simulink model "player_ball_7_8players"  (R2021b)
settings: Solver=VariableStepAuto  StartTime=0.0  StopTime=300  RelTol=1e-3
model workspace (MAT data in the model file):
  trailfuzzy = 'trailfuzzy.fis'
values from neighbouring files (symbols this model uses):
  initBallPos = fieldCenter    [robotSoccerParams.m]
  robotDetectorMaxHits = 5    [robotSoccerParams.m]
  sampleTime = 0.05    [robotSoccerParams.m]
undefined symbols (not defined in the file or in its folder): DiscIntNeverNeededParam
libraries: mobileRoboticsLib x41, dspindex x14, fuzblock x8
(part 2 of 2)

== matlab function player_ball_7_8players/idx3 goal_range_angles ==
  data: u input; goalRight_angle output; goalRange output; goalLeft_angle output; rPose_x input; rPose_y input
% function y = fcn(u)
% for i = 1:5
%     if u(i,3) == 1
%         a = u(i,:)
%     end
% end
% % b = u(2,:)
% % c = u(3,:)
% % d = u(4,:)
% % e = u(5,:)
% y = a;
% end
%two indexes are same. How to identify right and left angles
% for now randomly assigned the values
% goal range is minimum of the two 


function [goalRight_angle,goalRange, goalLeft_angle]= fcn(u,rPose_x, rPose_y)
goalRight_angle=0;
goalLeft_angle=0;
right_range = 0;
left_range =0;

x=0;
%if rPose_y1> 15 &&  rPose_y1< 45 && rPose_theta1 > 0
leftPolePose = [90 45];
rightPolePose = [90 15];
robotPose = [rPose_x rPose_y];
rightPole_dist = norm(rightPolePose - robotPose);
leftPole_dist = norm(leftPolePose - robotPose);
if rightPole_dist< leftPole_dist
    k=0;
    for i= 1:5
        if u(i,3) == 3 && k==0
            goalRight_angle = u(i,2);
            right_range = u(i,1);
            k = k+1;
        elseif u(i,3) ==3 && k==1
            goalLeft_angle = u(i,2);
            left_range = u(i,1);
            k =0;

        end
    end
else
    k=0;
    for i= 1:5
        if u(i,3) == 3 && k==0
            goalLeft_angle = u(i,2);
            left_range = u(i,1);
            k = k+1;
        elseif u(i,3) ==3 && k==1
            goalRight_angle = u(i,2);
            right_range = u(i,1);
            k =0;

        end
    end
end

if right_range < left_range
    goalRange = right_range;
else
    goalRange = left_range;
end

== matlab function player_ball_7_8players/Zero Pad Detections4 ==
  data: u input size=[maxHits 3]; y output size=[maxHits 3]; maxHits parameter
function y = zeroPad(u,maxHits)
% Zero-pads object detections to work with arrays of buses

y = zeros(maxHits,3);
numElems = min(size(u,1),maxHits);
for idx = 1:numElems
   y(idx,1:3) = u(idx,1:3); 
end

== matlab function player_ball_7_8players/Ball Dynamics1 ==
  data: ballPose output; ballHeld input; KickPower input; rPose_x input; rPose_y input; rPose_theta input
function ballPose  = fcn(ballHeld, KickPower,rPose_x, rPose_y, rPose_theta)
ballPose = [25 10];
if ballHeld == 1 
    ballPose = [rPose_x rPose_y] + (0.8 + 0.3)*[cos(rPose_theta) sin(rPose_theta)];

elseif KickPower >= 5.5 && ballHeld == 1
    %ballPose = KickPower*[rPose_x rPose_y] + (0.8 + 0.3)*[cos(rPose_theta) sin(rPose_theta)];
    ballHeld = 0
    ballPose = KickPower*[rPose_x rPose_y] + (0.8 + 0.3)*[cos(rPose_theta) sin(rPose_theta)];
    %if KickPower ~=0
    %    ballPose = KickPower*[rPose_x rPose_y] + (0.8 + 0.3)*[cos(rPose_theta) sin(rPose_theta)];
    %end

end

== matlab function player_ball_7_8players/MATLAB Function1 ==
  data: u input; y output
function y = fcn(u)

if u > 3.15
    u = pi -(u - pi);
end

if u <-3.15
    u = pi + (u + pi);
end     

y = u;

== matlab function player_ball_7_8players/Zero Pad Detections1 ==
  data: u input size=[maxHits 3]; y output size=[maxHits 3]; maxHits parameter
function y = zeroPad(u,maxHits)
% Zero-pads object detections to work with arrays of buses

y = zeros(maxHits,3);
numElems = min(size(u,1),maxHits);
for idx = 1:numElems
   y(idx,1:3) = u(idx,1:3); 
end

== matlab function player_ball_7_8players/Zero Pad Detections5 ==
  data: u input size=[maxHits 3]; y output size=[maxHits 3]; maxHits parameter
function y = zeroPad(u,maxHits)
% Zero-pads object detections to work with arrays of buses

y = zeros(maxHits,3);
numElems = min(size(u,1),maxHits);
for idx = 1:numElems
   y(idx,1:3) = u(idx,1:3); 
end

== matlab function player_ball_7_8players/Zero Pad Detections6 ==
  data: u input size=[maxHits 3]; y output size=[maxHits 3]; maxHits parameter
function y = zeroPad(u,maxHits)
% Zero-pads object detections to work with arrays of buses

y = zeros(maxHits,3);
numElems = min(size(u,1),maxHits);
for idx = 1:numElems
   y(idx,1:3) = u(idx,1:3); 
end

== matlab function player_ball_7_8players/Zero Pad Detections7 ==
  data: u input size=[maxHits 3]; y output size=[maxHits 3]; maxHits parameter
function y = zeroPad(u,maxHits)
% Zero-pads object detections to work with arrays of buses

y = zeros(maxHits,3);
numElems = min(size(u,1),maxHits);
for idx = 1:numElems
   y(idx,1:3) = u(idx,1:3); 
end

== matlab function player_ball_7_8players/ball1 ==
  data: u input; y output; ballHeld output; robotIdx output; ballHeld input; robotIdx input

function [y,ballHeld, robotIdx]= fcn(u,ballHeld,robotIdx)
% a = u(1,:);
% b = u(2,:);
% c = u(3,:);
% d = u(4,:);
% e = u(5,:);
% robotIdx =2;
% if a(3) ==1
%     y = a;
% 
% 
% elseif b(3) ==1
%     y = b;
% 
% 
% elseif c(3)==1
%     y=c;
% 
% 
% elseif d(3)==1
%     y=d;
% 
% 
% else
%     y = e;
% 
% 
% end
% if y(1)  <= 1.1
%     ballHeld = 1;
%     %robotIdx =2;
% 
% else
%     ballHeld =0;
%     %robotIdx =0;
% 
% end
a = u(1,:);
b = u(2,:);
c = u(3,:);
d = u(4,:);
e = u(5,:);
robotIdx =2;
if a(3) ==1
    y = a;


elseif b(3) ==1
    y = b;


elseif c(3)==1
    y=c;


elseif d(3)==1
    y=d;


else
    y = e;


end
if y(1)  <= 1.1
    ballHeld = 1;
    %robotIdx =1;
    %possession = robotIdx;

else
    ballHeld =0;
    %robotIdx =0;

end

== matlab function player_ball_7_8players/idx3 goal_range_angles1 ==
  data: u input; goalRight_angle output; goalRange output; goalLeft_angle output; rPose_x input; rPose_y input
% function y = fcn(u)
% for i = 1:5
%     if u(i,3) == 1
%         a = u(i,:)
%     end
% end
% % b = u(2,:)
% % c = u(3,:)
% % d = u(4,:)
% % e = u(5,:)
% y = a;
% end
%two indexes are same. How to identify right and left angles
% for now randomly assigned the values
% goal range is minimum of the two 


function [goalRight_angle,goalRange, goalLeft_angle]= fcn(u,rPose_x,rPose_y)
goalRight_angle=0;
goalLeft_angle=0;
right_range = 0;
left_range =0;

x=0;
%if rPose_y1> 15 &&  rPose_y1< 45 && rPose_theta1 > 0
leftPolePose = [90 45];
rightPolePose = [90 15];
robotPose = [rPose_x rPose_y];
rightPole_dist = norm(rightPolePose - robotPose);
leftPole_dist = norm(leftPolePose - robotPose);
if rightPole_dist< leftPole_dist
    k=0;
    for i= 1:5
        if u(i,3) == 3 && k==0
            goalRight_angle = u(i,2);
            right_range = u(i,1);
            k = k+1;
        elseif u(i,3) ==3 && k==1
            goalLeft_angle = u(i,2);
            left_range = u(i,1);
            k =0;

        end
    end
else
    k=0;
    for i= 1:5
        if u(i,3) == 3 && k==0
            goalLeft_angle = u(i,2);
            left_range = u(i,1);
            k = k+1;
        elseif u(i,3) ==3 && k==1
            goalRight_angle = u(i,2);
            right_range = u(i,1);
            k =0;

        end
    end
end

if right_range < left_range
    goalRange = right_range;
else
    goalRange = left_range;
end

== matlab function player_ball_7_8players/Zero Pad Detections8 ==
  data: u input size=[maxHits 3]; y output size=[maxHits 3]; maxHits parameter
function y = zeroPad(u,maxHits)
% Zero-pads object detections to work with arrays of buses

y = zeros(maxHits,3);
numElems = min(size(u,1),maxHits);
for idx = 1:numElems
   y(idx,1:3) = u(idx,1:3); 
end

== matlab function player_ball_7_8players/Zero Pad Detections9 ==
  data: u input size=[maxHits 3]; y output size=[maxHits 3]; maxHits parameter
function y = zeroPad(u,maxHits)
% Zero-pads object detections to work with arrays of buses

y = zeros(maxHits,3);
numElems = min(size(u,1),maxHits);
for idx = 1:numElems
   y(idx,1:3) = u(idx,1:3); 
end

== stateflow chart player_ball_7_8players/Chart3 ==
  state ballDynamics [parallel]
    en:
    coder.extrinsic('randn');
    setBallState([45 30],0,0);
    settings: executionOrder=2
    state InBounds
      en:
      randNum = randn(2,1);
      state BallFree
      state BallHeld
        en,du:
        ballPose = [rPose_X rPose_Y] + ...
        (0.8+0.3)*[cos(rPose_Theta) sin(rPose_Theta)];
      (default) -> BallFree
      BallHeld -> BallFree : [kickPower>2]{setBallState(ballPose,kickPower*3+BallVel, ...
          |  rPose_Theta),possession =0}
      BallFree -> BallHeld : [after(2,sec) && ...
          |  ballheld > 0]
    state Outofbounds
      en:
      ballPose = [45 30];
      setBallState(ballPose,0,rPose_Theta)
    (default) -> InBounds
    Outofbounds -> InBounds : [after(1,sec)]
    InBounds -> Outofbounds : [ballPose(1) > 90 || ballPose(2) > 60 || ballPose(1) < 0 || ballPose(2) < 0]
  state Posession [parallel]
    en:
    possession=0;
    ballheld =0;
    du:
    %possession=0;
    for i=1:8
    if ballHeld(i) == 1
    possession = i
    % else
    % possession = 0;
    end
    end
    if possession ~=0
    rPose_X = rPose_x(possession);
    rPose_Y = rPose_y(possession);
    rPose_Theta = rPose_theta(possession);
    kickPower = KickPower(possession);
    BallVel = ballVel(possession);
    ballheld = ballHeld(possession)
    if ballheld == 0
    %   teamHeld = 1;
    % else
    teamHeld = 0
    possession = 0
    end
    if possession == 1 || possession == 2 || possession ==3 || possession == 4
    teamHeld = 1
    elseif possession ==5 || possession == 6 || possession == 7 || possession ==8
    teamHeld = 2
    end
    %else
    %rPose_X= 0;
    %rPose_Y =0;
    %rPose_Theta = 0;
    %kickPower = 0;
    % BallVel = 0;
    % ballheld = 0;
    %teamHeld =0;
    end
    settings: executionOrder=1
  state setBallState(pos,vel,theta) [function]
  data: sf_internal_action_state_placeholder_data local double size=1 =0; pos function_input double size=[1 2]; vel function_input double size=1; theta function_input double size=1; ballHeld input; KickPower input; rPose_x input; rPose_y input; rPose_theta input; robotIdx input; ballPose output; randNum local; action local; ballVel input; i local; possession local; BallVel local; ballheld local; kickPower local; rPose_Theta local; rPose_X local; rPose_Y local; teamHeld output

== matlab function player_ball_7_8players/ball3 ==
  data: u input; y output; ballHeld output; robotIdx output; ballHeld input; robotIdx input

function [y,ballHeld, robotIdx]= fcn(u,ballHeld,robotIdx)
a = u(1,:);
b = u(2,:);
c = u(3,:);
d = u(4,:);
e = u(5,:);
robotIdx =3;
if a(3) ==1
    y = a;


elseif b(3) ==1
    y = b;


elseif c(3)==1
    y=c;


elseif d(3)==1
    y=d;


else
    y = e;


end
if y(1)  <= 1.1
    ballHeld = 1;
    %robotIdx =1;
    %possession = robotIdx;

else
    ballHeld =0;
    %robotIdx =0;

end

== matlab function player_ball_7_8players/idx3 goal_range_angles3 ==
  data: u input; goalRight_angle output; goalRange output; goalLeft_angle output; rPose_x input; rPose_y input
% function y = fcn(u)
% for i = 1:5
%     if u(i,3) == 1
%         a = u(i,:)
%     end
% end
% % b = u(2,:)
% % c = u(3,:)
% % d = u(4,:)
% % e = u(5,:)
% y = a;
% end
%two indexes are same. How to identify right and left angles
% for now randomly assigned the values
% goal range is minimum of the two 


function [goalRight_angle,goalRange, goalLeft_angle]= fcn(u,rPose_x, rPose_y)
goalRight_angle=0;
goalLeft_angle=0;
right_range = 0;
left_range =0;

x=0;
%if rPose_y1> 15 &&  rPose_y1< 45 && rPose_theta1 > 0
leftPolePose = [90 45];
rightPolePose = [90 15];
robotPose = [rPose_x rPose_y];
rightPole_dist = norm(rightPolePose - robotPose);
leftPole_dist = norm(leftPolePose - robotPose);
if rightPole_dist< leftPole_dist
    k=0;
    for i= 1:5
        if u(i,3) == 3 && k==0
            goalRight_angle = u(i,2);
            right_range = u(i,1);
            k = k+1;
        elseif u(i,3) ==3 && k==1
            goalLeft_angle = u(i,2);
            left_range = u(i,1);
            k =0;

        end
    end
else
    k=0;
    for i= 1:5
        if u(i,3) == 3 && k==0
            goalLeft_angle = u(i,2);
            left_range = u(i,1);
            k = k+1;
        elseif u(i,3) ==3 && k==1
            goalRight_angle = u(i,2);
            right_range = u(i,1);
            k =0;

        end
    end
end

if right_range < left_range
    goalRange = right_range;
else
    goalRange = left_range;
end

== matlab function player_ball_7_8players/Zero Pad Detections10 ==
  data: u input size=[maxHits 3]; y output size=[maxHits 3]; maxHits parameter
function y = zeroPad(u,maxHits)
% Zero-pads object detections to work with arrays of buses

y = zeros(maxHits,3);
numElems = min(size(u,1),maxHits);
for idx = 1:numElems
   y(idx,1:3) = u(idx,1:3); 
end

== matlab function player_ball_7_8players/Zero Pad Detections11 ==
  data: u input size=[maxHits 3]; y output size=[maxHits 3]; maxHits parameter
function y = zeroPad(u,maxHits)
% Zero-pads object detections to work with arrays of buses

y = zeros(maxHits,3);
numElems = min(size(u,1),maxHits);
for idx = 1:numElems
   y(idx,1:3) = u(idx,1:3); 
end

== matlab function player_ball_7_8players/Zero Pad Detections12 ==
  data: u input size=[maxHits 3]; y output size=[maxHits 3]; maxHits parameter
function y = zeroPad(u,maxHits)
% Zero-pads object detections to work with arrays of buses

y = zeros(maxHits,3);
numElems = min(size(u,1),maxHits);
for idx = 1:numElems
   y(idx,1:3) = u(idx,1:3); 
end

== matlab function player_ball_7_8players/ball4 ==
  data: u input; y output; ballHeld output; robotIdx output; ballHeld input; robotIdx input

function [y,ballHeld, robotIdx]= fcn(u,ballHeld,robotIdx)
% a = u(1,:);
% b = u(2,:);
% c = u(3,:);
% d = u(4,:);
% e = u(5,:);
% robotIdx =2;
% if a(3) ==1
%     y = a;
% 
% 
% elseif b(3) ==1
%     y = b;
% 
% 
% elseif c(3)==1
%     y=c;
% 
% 
% elseif d(3)==1
%     y=d;
% 
% 
% else
%     y = e;
% 
% 
% end
% if y(1)  <= 1.1
%     ballHeld = 1;
%     %robotIdx =2;
% 
% else
%     ballHeld =0;
%     %robotIdx =0;
% 
% end
a = u(1,:);
b = u(2,:);
c = u(3,:);
d = u(4,:);
e = u(5,:);
robotIdx =4;
if a(3) ==1
    y = a;


elseif b(3) ==1
    y = b;


elseif c(3)==1
    y=c;


elseif d(3)==1
    y=d;


else
    y = e;


end
if y(1)  <= 1.1
    ballHeld = 1;
    %robotIdx =1;
    %possession = robotIdx;

else
    ballHeld =0;
    %robotIdx =0;

end

== matlab function player_ball_7_8players/idx3 goal_range_angles4 ==
  data: u input; goalRight_angle output; goalRange output; goalLeft_angle output; rPose_x input; rPose_y input
% function y = fcn(u)
% for i = 1:5
%     if u(i,3) == 1
%         a = u(i,:)
%     end
% end
% % b = u(2,:)
% % c = u(3,:)
% % d = u(4,:)
% % e = u(5,:)
% y = a;
% end
%two indexes are same. How to identify right and left angles
% for now randomly assigned the values
% goal range is minimum of the two 


function [goalRight_angle,goalRange, goalLeft_angle]= fcn(u,rPose_x,rPose_y)
goalRight_angle=0;
goalLeft_angle=0;
right_range = 0;
left_range =0;

x=0;
%if rPose_y1> 15 &&  rPose_y1< 45 && rPose_theta1 > 0
leftPolePose = [90 45];
rightPolePose = [90 15];
robotPose = [rPose_x rPose_y];
rightPole_dist = norm(rightPolePose - robotPose);
leftPole_dist = norm(leftPolePose - robotPose);
if rightPole_dist< leftPole_dist
    k=0;
    for i= 1:5
        if u(i,3) == 3 && k==0
            goalRight_angle = u(i,2);
            right_range = u(i,1);
            k = k+1;
        elseif u(i,3) ==3 && k==1
            goalLeft_angle = u(i,2);
            left_range = u(i,1);
            k =0;

        end
    end
else
    k=0;
    for i= 1:5
        if u(i,3) == 3 && k==0
            goalLeft_angle = u(i,2);
            left_range = u(i,1);
            k = k+1;
        elseif u(i,3) ==3 && k==1
            goalRight_angle = u(i,2);
            right_range = u(i,1);
            k =0;

        end
    end
end

if right_range < left_range
    goalRange = right_range;
else
    goalRange = left_range;
end

== matlab function player_ball_7_8players/Ball Dynamics2 ==
  data: ballPose output; ballHeld input; KickPower input; rPose_x input; rPose_y input; rPose_theta input
function ballPose  = fcn(ballHeld, KickPower,rPose_x, rPose_y, rPose_theta)
ballPose = [25 10];
if ballHeld == 1 
    ballPose = [rPose_x rPose_y] + (0.8 + 0.3)*[cos(rPose_theta) sin(rPose_theta)];

elseif KickPower >= 5.5 && ballHeld == 1
    %ballPose = KickPower*[rPose_x rPose_y] + (0.8 + 0.3)*[cos(rPose_theta) sin(rPose_theta)];
    ballHeld = 0
    ballPose = KickPower*[rPose_x rPose_y] + (0.8 + 0.3)*[cos(rPose_theta) sin(rPose_theta)];
    %if KickPower ~=0
    %    ballPose = KickPower*[rPose_x rPose_y] + (0.8 + 0.3)*[cos(rPose_theta) sin(rPose_theta)];
    %end

end

== matlab function player_ball_7_8players/Ball Dynamics3 ==
  data: ballPose output; ballHeld input; KickPower input; rPose_x input; rPose_y input; rPose_theta input
function ballPose  = fcn(ballHeld, KickPower,rPose_x, rPose_y, rPose_theta)
ballPose = [25 10];
if ballHeld == 1 
    ballPose = [rPose_x rPose_y] + (0.8 + 0.3)*[cos(rPose_theta) sin(rPose_theta)];

elseif KickPower >= 5.5 && ballHeld == 1
    %ballPose = KickPower*[rPose_x rPose_y] + (0.8 + 0.3)*[cos(rPose_theta) sin(rPose_theta)];
    ballHeld = 0
    ballPose = KickPower*[rPose_x rPose_y] + (0.8 + 0.3)*[cos(rPose_theta) sin(rPose_theta)];
    %if KickPower ~=0
    %    ballPose = KickPower*[rPose_x rPose_y] + (0.8 + 0.3)*[cos(rPose_theta) sin(rPose_theta)];
    %end

end

== matlab function player_ball_7_8players/MATLAB Function2 ==
  data: u input; y output
function y = fcn(u)

if u > 3.15
    u = pi -(u - pi);
end

if u <-3.15
    u = pi + (u + pi);
end     

y = u;

== matlab function player_ball_7_8players/MATLAB Function3 ==
  data: u input; y output
function y = fcn(u)

if u > 3.15
    u = pi -(u - pi);
end

if u <-3.15
    u = pi + (u + pi);
end     

y = u;

== matlab function player_ball_7_8players/Zero Pad Detections13 ==
  data: u input size=[maxHits 3]; y output size=[maxHits 3]; maxHits parameter
function y = zeroPad(u,maxHits)
% Zero-pads object detections to work with arrays of buses

y = zeros(maxHits,3);
numElems = min(size(u,1),maxHits);
for idx = 1:numElems
   y(idx,1:3) = u(idx,1:3); 
end

== matlab function player_ball_7_8players/Zero Pad Detections14 ==
  data: u input size=[maxHits 3]; y output size=[maxHits 3]; maxHits parameter
function y = zeroPad(u,maxHits)
% Zero-pads object detections to work with arrays of buses

y = zeros(maxHits,3);
numElems = min(size(u,1),maxHits);
for idx = 1:numElems
   y(idx,1:3) = u(idx,1:3); 
end

== matlab function player_ball_7_8players/Zero Pad Detections15 ==
  data: u input size=[maxHits 3]; y output size=[maxHits 3]; maxHits parameter
function y = zeroPad(u,maxHits)
% Zero-pads object detections to work with arrays of buses

y = zeros(maxHits,3);
numElems = min(size(u,1),maxHits);
for idx = 1:numElems
   y(idx,1:3) = u(idx,1:3); 
end

== matlab function player_ball_7_8players/Zero Pad Detections16 ==
  data: u input size=[maxHits 3]; y output size=[maxHits 3]; maxHits parameter
function y = zeroPad(u,maxHits)
% Zero-pads object detections to work with arrays of buses

y = zeros(maxHits,3);
numElems = min(size(u,1),maxHits);
for idx = 1:numElems
   y(idx,1:3) = u(idx,1:3); 
end

== matlab function player_ball_7_8players/Zero Pad Detections17 ==
  data: u input size=[maxHits 3]; y output size=[maxHits 3]; maxHits parameter
function y = zeroPad(u,maxHits)
% Zero-pads object detections to work with arrays of buses

y = zeros(maxHits,3);
numElems = min(size(u,1),maxHits);
for idx = 1:numElems
   y(idx,1:3) = u(idx,1:3); 
end

== matlab function player_ball_7_8players/Zero Pad Detections18 ==
  data: u input size=[maxHits 3]; y output size=[maxHits 3]; maxHits parameter
function y = zeroPad(u,maxHits)
% Zero-pads object detections to work with arrays of buses

y = zeros(maxHits,3);
numElems = min(size(u,1),maxHits);
for idx = 1:numElems
   y(idx,1:3) = u(idx,1:3); 
end

== matlab function player_ball_7_8players/Zero Pad Detections19 ==
  data: u input size=[maxHits 3]; y output size=[maxHits 3]; maxHits parameter
function y = zeroPad(u,maxHits)
% Zero-pads object detections to work with arrays of buses

y = zeros(maxHits,3);
numElems = min(size(u,1),maxHits);
for idx = 1:numElems
   y(idx,1:3) = u(idx,1:3); 
end

== matlab function player_ball_7_8players/Zero Pad Detections20 ==
  data: u input size=[maxHits 3]; y output size=[maxHits 3]; maxHits parameter
function y = zeroPad(u,maxHits)
% Zero-pads object detections to work with arrays of buses

y = zeros(maxHits,3);
numElems = min(size(u,1),maxHits);
for idx = 1:numElems
   y(idx,1:3) = u(idx,1:3); 
end

== matlab function player_ball_7_8players/Zero Pad Detections21 ==
  data: u input size=[maxHits 3]; y output size=[maxHits 3]; maxHits parameter
function y = zeroPad(u,maxHits)
% Zero-pads object detections to work with arrays of buses

y = zeros(maxHits,3);
numElems = min(size(u,1),maxHits);
for idx = 1:numElems
   y(idx,1:3) = u(idx,1:3); 
end

== matlab function player_ball_7_8players/Zero Pad Detections22 ==
  data: u input size=[maxHits 3]; y output size=[maxHits 3]; maxHits parameter
function y = zeroPad(u,maxHits)
% Zero-pads object detections to work with arrays of buses

y = zeros(maxHits,3);
numElems = min(size(u,1),maxHits);
for idx = 1:numElems
   y(idx,1:3) = u(idx,1:3); 
end

== matlab function player_ball_7_8players/Zero Pad Detections23 ==
  data: u input size=[maxHits 3]; y output size=[maxHits 3]; maxHits parameter
function y = zeroPad(u,maxHits)
% Zero-pads object detections to work with arrays of buses

y = zeros(maxHits,3);
numElems = min(size(u,1),maxHits);
for idx = 1:numElems
   y(idx,1:3) = u(idx,1:3); 
end

== matlab function player_ball_7_8players/Zero Pad Detections24 ==
  data: u input size=[maxHits 3]; y output size=[maxHits 3]; maxHits parameter
function y = zeroPad(u,maxHits)
% Zero-pads object detections to work with arrays of buses

y = zeros(maxHits,3);
numElems = min(size(u,1),maxHits);
for idx = 1:numElems
   y(idx,1:3) = u(idx,1:3); 
end

== matlab function player_ball_7_8players/ball2 ==
  data: u input; y output; ballHeld output; robotIdx output; ballHeld input; robotIdx input

function [y,ballHeld, robotIdx]= fcn(u,ballHeld,robotIdx)
a = u(1,:);
b = u(2,:);
c = u(3,:);
d = u(4,:);
e = u(5,:);
robotIdx =5;
if a(3) ==1
    y = a;


elseif b(3) ==1
    y = b;


elseif c(3)==1
    y=c;


elseif d(3)==1
    y=d;


else
    y = e;


end
if y(1)  <= 1.1
    ballHeld = 1;
    %robotIdx =1;
    %possession = robotIdx;

else
    ballHeld =0;
    %robotIdx =0;

end

== matlab function player_ball_7_8players/ball5 ==
  data: u input; y output; ballHeld output; robotIdx output; ballHeld input; robotIdx input

function [y,ballHeld, robotIdx]= fcn(u,ballHeld,robotIdx)
% a = u(1,:);
% b = u(2,:);
% c = u(3,:);
% d = u(4,:);
% e = u(5,:);
% robotIdx =2;
% if a(3) ==1
%     y = a;
% 
% 
% elseif b(3) ==1
%     y = b;
% 
% 
% elseif c(3)==1
%     y=c;
% 
% 
% elseif d(3)==1
%     y=d;
% 
% 
% else
%     y = e;
% 
% 
% end
% if y(1)  <= 1.1
%     ballHeld = 1;
%     %robotIdx =2;
% 
% else
%     ballHeld =0;
%     %robotIdx =0;
% 
% end
a = u(1,:);
b = u(2,:);
c = u(3,:);
d = u(4,:);
e = u(5,:);
robotIdx =6;
if a(3) ==1
    y = a;


elseif b(3) ==1
    y = b;


elseif c(3)==1
    y=c;


elseif d(3)==1
    y=d;


else
    y = e;


end
if y(1)  <= 1.1
    ballHeld = 1;
    %robotIdx =1;
    %possession = robotIdx;

else
    ballHeld =0;
    %robotIdx =0;

end

== matlab function player_ball_7_8players/ball6 ==
  data: u input; y output; ballHeld output; robotIdx output; ballHeld input; robotIdx input

function [y,ballHeld, robotIdx]= fcn(u,ballHeld,robotIdx)
a = u(1,:);
b = u(2,:);
c = u(3,:);
d = u(4,:);
e = u(5,:);
robotIdx =7;
if a(3) ==1
    y = a;


elseif b(3) ==1
    y = b;


elseif c(3)==1
    y=c;


elseif d(3)==1
    y=d;


else
    y = e;


end
if y(1)  <= 1.1
    ballHeld = 1;
    %robotIdx =1;
    %possession = robotIdx;

else
    ballHeld =0;
    %robotIdx =0;

end

== matlab function player_ball_7_8players/ball7 ==
  data: u input; y output; ballHeld output; robotIdx output; ballHeld input; robotIdx input

function [y,ballHeld, robotIdx]= fcn(u,ballHeld,robotIdx)
% a = u(1,:);
% b = u(2,:);
% c = u(3,:);
% d = u(4,:);
% e = u(5,:);
% robotIdx =8;
% if a(3) ==1
%     y = a;
% 
% 
% elseif b(3) ==1
%     y = b;
% 
% 
% elseif c(3)==1
%     y=c;
% 
% 
% elseif d(3)==1
%     y=d;
% 
% 
% else
%     y = e;
% 
% 
% end
% if y(1)  <= 1.1
%     ballHeld = 1;
%     %robotIdx =2;
% 
% else
%     ballHeld =0;
%     %robotIdx =0;
% 
% end
a = u(1,:);
b = u(2,:);
c = u(3,:);
d = u(4,:);
e = u(5,:);
robotIdx =8;
if a(3) ==1
    y = a;


elseif b(3) ==1
    y = b;


elseif c(3)==1
    y=c;


elseif d(3)==1
    y=d;


else
    y = e;


end
if y(1)  <= 1.1
    ballHeld = 1;
    %robotIdx =1;
    %possession = robotIdx;

else
    ballHeld =0;
    %robotIdx =0;

end

== matlab function player_ball_7_8players/idx3 goal_range_angles2 ==
  data: u input; goalRight_angle output; goalRange output; goalLeft_angle output; rPose_x input; rPose_y input
% function y = fcn(u)
% for i = 1:5
%     if u(i,3) == 1
%         a = u(i,:)
%     end
% end
% % b = u(2,:)
% % c = u(3,:)
% % d = u(4,:)
% % e = u(5,:)
% y = a;
% end
%two indexes are same. How to identify right and left angles
% for now randomly assigned the values
% goal range is minimum of the two 


function [goalRight_angle,goalRange, goalLeft_angle]= fcn(u,rPose_x, rPose_y)
goalRight_angle=0;
goalLeft_angle=0;
right_range = 0;
left_range =0;

x=0;
%if rPose_y1> 15 &&  rPose_y1< 45 && rPose_theta1 > 0
leftPolePose = [0 45];
rightPolePose = [0 15];
robotPose = [rPose_x rPose_y];
rightPole_dist = norm(rightPolePose - robotPose);
leftPole_dist = norm(leftPolePose - robotPose);
if rightPole_dist< leftPole_dist
    k=0;
    for i= 1:5
        if u(i,3) == 2 && k==0
            goalRight_angle = u(i,2);
            right_range = u(i,1);
            k = k+1;
        elseif u(i,3) ==2 && k==1
            goalLeft_angle = u(i,2);
            left_range = u(i,1);
            k =0;

        end
    end
else
    k=0;
    for i= 1:5
        if u(i,3) == 2 && k==0
            goalLeft_angle = u(i,2);
            left_range = u(i,1);
            k = k+1;
        elseif u(i,3) ==2 && k==1
            goalRight_angle = u(i,2);
            right_range = u(i,1);
            k =0;

        end
    end
end

if right_range < left_range
    goalRange = right_range;
else
    goalRange = left_range;
end

== matlab function player_ball_7_8players/idx3 goal_range_angles5 ==
  data: u input; goalRight_angle output; goalRange output; goalLeft_angle output; rPose_x input; rPose_y input
% function y = fcn(u)
% for i = 1:5
%     if u(i,3) == 1
%         a = u(i,:)
%     end
% end
% % b = u(2,:)
% % c = u(3,:)
% % d = u(4,:)
% % e = u(5,:)
% y = a;
% end
%two indexes are same. How to identify right and left angles
% for now randomly assigned the values
% goal range is minimum of the two 


function [goalRight_angle,goalRange, goalLeft_angle]= fcn(u,rPose_x,rPose_y)
goalRight_angle=0;
goalLeft_angle=0;
right_range = 0;
left_range =0;

x=0;
%if rPose_y1> 15 &&  rPose_y1< 45 && rPose_theta1 > 0
leftPolePose = [0 45];
rightPolePose = [0 15];
robotPose = [rPose_x rPose_y];
rightPole_dist = norm(rightPolePose - robotPose);
leftPole_dist = norm(leftPolePose - robotPose);
if rightPole_dist< leftPole_dist
    k=0;
    for i= 1:5
        if u(i,3) == 2 && k==0
            goalRight_angle = u(i,2);
            right_range = u(i,1);
            k = k+1;
        elseif u(i,3) ==2 && k==1
            goalLeft_angle = u(i,2);
            left_range = u(i,1);
            k =0;

        end
    end
else
    k=0;
    for i= 1:5
        if u(i,3) == 2 && k==0
            goalLeft_angle = u(i,2);
            left_range = u(i,1);
            k = k+1;
        elseif u(i,3) ==2 && k==1
            goalRight_angle = u(i,2);
            right_range = u(i,1);
            k =0;

        end
    end
end

if right_range < left_range
    goalRange = right_range;
else
    goalRange = left_range;
end

== matlab function player_ball_7_8players/idx3 goal_range_angles6 ==
  data: u input; goalRight_angle output; goalRange output; goalLeft_angle output; rPose_x input; rPose_y input
% function y = fcn(u)
% for i = 1:5
%     if u(i,3) == 1
%         a = u(i,:)
%     end
% end
% % b = u(2,:)
% % c = u(3,:)
% % d = u(4,:)
% % e = u(5,:)
% y = a;
% end
%two indexes are same. How to identify right and left angles
% for now randomly assigned the values
% goal range is minimum of the two 


function [goalRight_angle,goalRange, goalLeft_angle]= fcn(u,rPose_x, rPose_y)
goalRight_angle=0;
goalLeft_angle=0;
right_range = 0;
left_range =0;

x=0;
%if rPose_y1> 15 &&  rPose_y1< 45 && rPose_theta1 > 0
leftPolePose = [0 45];
rightPolePose = [0 15];
robotPose = [rPose_x rPose_y];
rightPole_dist = norm(rightPolePose - robotPose);
leftPole_dist = norm(leftPolePose - robotPose);
if rightPole_dist< leftPole_dist
    k=0;
    for i= 1:5
        if u(i,3) == 2 && k==0
            goalRight_angle = u(i,2);
            right_range = u(i,1);
            k = k+1;
        elseif u(i,3) ==2 && k==1
            goalLeft_angle = u(i,2);
            left_range = u(i,1);
            k =0;

        end
    end
else
    k=0;
    for i= 1:5
        if u(i,3) == 2 && k==0
            goalLeft_angle = u(i,2);
            left_range = u(i,1);
            k = k+1;
        elseif u(i,3) ==2 && k==1
            goalRight_angle = u(i,2);
            right_range = u(i,1);
            k =0;

        end
    end
end

if right_range < left_range
    goalRange = right_range;
else
    goalRange = left_range;
end

== matlab function player_ball_7_8players/idx3 goal_range_angles7 ==
  data: u input; goalRight_angle output; goalRange output; goalLeft_angle output; rPose_x input; rPose_y input
% function y = fcn(u)
% for i = 1:5
%     if u(i,3) == 1
%         a = u(i,:)
%     end
% end
% % b = u(2,:)
% % c = u(3,:)
% % d = u(4,:)
% % e = u(5,:)
% y = a;
% end
%two indexes are same. How to identify right and left angles
% for now randomly assigned the values
% goal range is minimum of the two 


function [goalRight_angle,goalRange, goalLeft_angle]= fcn(u,rPose_x,rPose_y)
goalRight_angle=0;
goalLeft_angle=0;
right_range = 0;
left_range =0;

x=0;
%if rPose_y1> 15 &&  rPose_y1< 45 && rPose_theta1 > 0
leftPolePose = [0 45];
rightPolePose = [0 15];
robotPose = [rPose_x rPose_y];
rightPole_dist = norm(rightPolePose - robotPose);
leftPole_dist = norm(leftPolePose - robotPose);
if rightPole_dist< leftPole_dist
    k=0;
    for i= 1:5
        if u(i,3) == 2 && k==0
            goalRight_angle = u(i,2);
            right_range = u(i,1);
            k = k+1;
        elseif u(i,3) ==2 && k==1
            goalLeft_angle = u(i,2);
            left_range = u(i,1);
            k =0;

        end
    end
else
    k=0;
    for i= 1:5
        if u(i,3) == 2 && k==0
            goalLeft_angle = u(i,2);
            left_range = u(i,1);
            k = k+1;
        elseif u(i,3) ==2 && k==1
            goalRight_angle = u(i,2);
            right_range = u(i,1);
            k =0;

        end
    end
end

if right_range < left_range
    goalRange = right_range;
else
    goalRange = left_range;
end
